simulink model "Project_Mobius"  (R2023b)
settings: Solver=ode4  StartTime=0.0  StopTime=100  FixedStep=5e-3  RelTol=1e-3
values from neighbouring files (symbols this model uses):
  aileron_stuck = 0.1    [fault_insertion.m]
  aircraft_b = 2    [initial.m]
  aircraft_c = 0.275    [initial.m]
  aircraft_mass = 6.031    [initial.m]
  c1 = ((Iyy - Izz)*Izz - Ixz*Ixz)/sigma    (= -0.404494382022)    [initial.m]
  c2 = ((Ixx - Iyy + Izz)*Ixz)/sigma    (= 0)    [initial.m]
  c3 = Izz/sigma    (= 3.74531835206)    [initial.m]
  c4 = Ixz/sigma    (= 0)    [initial.m]
  c5 = (Izz - Ixx)/Iyy    (= 0.404494382022)    [initial.m]
  c6 = Ixz/Iyy    (= 0)    [initial.m]
  c7 = 1/Iyy    (= 3.74531835206)    [initial.m]
  c8 = (Ixx*(Ixx - Iyy) + Ixz*Ixz)/sigma    (= 0)    [initial.m]
  c9 = Ixx/sigma    (= 2.66666666667)    [initial.m]
  CD_fuselage = 0.027    [initial.m]
  CdDa = 0.092132    [initial.m]
  CdDe = 0.016043    [initial.m]
  CdDr = 0.0097403    [initial.m]
  CDmin = 0.06047    [initial.m]
  CL0 = 0.81857    [initial.m]
  CL_CDmin = 0.4806    [initial.m]
  CLa = 4.09127    [initial.m]
  CLa_dot = 0    [initial.m]
  Clb = -0.00161    [initial.m]
  ClDa = 0.286593    [initial.m]
  CLDa = -0.85291    [initial.m]
  CLDe = 0.50787    [initial.m]
  ClDr = 0.013407    [initial.m]
  Clp = -0.47584    [initial.m]
  CLq = 7.31097    [initial.m]
  Clr = 0.27153    [initial.m]
  Cm0 = 0.00763    [initial.m]
  Cma = -1.76966    [initial.m]
  CmDe = -1.83747    [initial.m]
  Cmq = -19.22663    [initial.m]
  Cnb = 0.0918    [initial.m]
  CnDa = 0.0049274    [initial.m]
  CnDr = -0.067036    [initial.m]
  Cnp = -0.13267    [initial.m]
  Cnr = -0.08829    [initial.m]
  CYb = -0.00157    [initial.m]
  CYDr = 0.128915    [initial.m]
  CYp = -0.00157    [initial.m]
  CYr = 0.18368    [initial.m]
  elevator_stuck = 0    [fault_insertion.m]
  fault_time_start = 1    [fault_insertion.m]
  flight_mode = 1    [initial.m]
  g = 9.8060    (= 9.806)    [initial.m]
  init_alpha = alpha_trim    (= 0)    [initial.m]
  init_h = 10    [initial.m]
  init_p = 0    [initial.m]
  init_phi = 0    [initial.m]
  init_psi = 0    [initial.m]
  init_q = 0    [initial.m]
  init_r = 0    [initial.m]
  init_theta = init_alpha    (= 0)    [initial.m]
  init_u = Vb(1)    [initial.m]
  init_v = Vb(2)    [initial.m]
  init_w = Vb(3)    [initial.m]
  init_x = 0    [initial.m]
  init_y = 0    [initial.m]
  K = 0.1328    [initial.m]
  Max_RPM = 10000    [initial.m]
  p_sensor_fault = 0    [fault_insertion.m]
  phi_sensor_fault = 0    [fault_insertion.m]
  PropDiameter = 0.3052    [initial.m]
  psi_sensor_fault = 0    [fault_insertion.m]
  q_sensor_fault = 0    [fault_insertion.m]
  r_sensor_fault = 0    [fault_insertion.m]
  rho = 1.2250    (= 1.225)    [initial.m]
  rotor1_direction = 1    [initial.m]
  rotor1_fail = 0    [fault_insertion.m]
  rotor2_direction = -1    [initial.m]
  rotor2_fail = 0    [fault_insertion.m]
  rotor3_direction = -1    [initial.m]
  rotor3_fail = 0    [fault_insertion.m]
  rotor4_direction = 1    [initial.m]
  rotor4_fail = 0    [fault_insertion.m]
  rotor_arm1 = [0.375,0.375,0]    [initial.m]
  rotor_arm2 = [0.375,-0.375,0]    [initial.m]
  rotor_arm3 = [-0.375,-0.375,0]    [initial.m]
  rotor_arm4 = [-0.375,0.375,0]    [initial.m]
  RPM1_init = rotor_n * 60    (= 5940)    [initial.m]
  RPM2_init = rotor_n * 60    (= 5940)    [initial.m]
  RPM3_init = 0    [initial.m]
  RPM4_init = 0    [initial.m]
  rudder_stuck = 0    [fault_insertion.m]
  theta_sensor_fault = 0    [fault_insertion.m]
  tilt1_fail = 0    [fault_insertion.m]
  tilt1_init = lambda    [initial.m]
  tilt2_fail = 0    [fault_insertion.m]
  tilt2_init = lambda    [initial.m]
  tilt3_init = 0    [initial.m]
  tilt4_init = 0    [initial.m]
  u_sensor_fault = 0    [fault_insertion.m]
  v_sensor_fault = 0    [fault_insertion.m]
  w_sensor_fault = 0    [fault_insertion.m]
undefined symbols (not defined in the file or in its folder): FixedWingMission, HoverMission
libraries: slpidlib x20, simulink_extras x12, simulink x7, aerolibasang x6, matrix_library x4, uavalgslib x4, sharedutil x1, sharedtransform x1
(part 4 of 4)

== system Project_Mobius/EVTOL Model/6DOF Dynamics/Subsystem ==
  In2 : Inport  Unit=rad  PortDimensions=3
  Create 3x3 Matrix : sharedutil/Create 3x3 Matrix  aMode=aMode
  Dead Zone : DeadZone  LowerValue=-cos(pi/2)  UpperValue=cos(pi/2)
  Fcn11 : Fcn  Expr=u(5)*u(4)
  Fcn12 : Fcn  Expr=u(5)*u(1)
  Fcn13 : Fcn  Expr=-u(2)
  Fcn21 : Fcn  Expr=u(3)*u(2)*u(4) - u(6)*u(1)
  Fcn22 : Fcn  Expr=u(3)*u(2)*u(1) + u(6)*u(4)
  Fcn23 : Fcn  Expr=u(3)*u(5)
  Fcn31 : Fcn  Expr=u(6)*u(2)*u(4) + u(3)*u(1)
  Fcn32 : Fcn  Expr=u(6)*u(2)*u(1) - u(3)*u(4)
  Fcn33 : Fcn  Expr=u(6)*u(5)
  Mux : Mux  Inputs=2
  sincos : Trigonometry  Operator=sincos
  DCMbe : Outport  Unit=1  PortDimensions=[3,3]  VectorParamsAs1DForOutWhenUnconnected=off
  wires:
  Fcn23/1 -> Create 3x3 Matrix/6
  Fcn31/1 -> Create 3x3 Matrix/7
  sincos/2 -> Dead Zone/1
  Fcn22/1 -> Create 3x3 Matrix/5
  Fcn21/1 -> Create 3x3 Matrix/4
  Fcn32/1 -> Create 3x3 Matrix/8
  Fcn33/1 -> Create 3x3 Matrix/9
  Mux/1 -> Fcn11/1, Fcn12/1, Fcn13/1, Fcn21/1, Fcn32/1, Fcn33/1, Fcn31/1, Fcn23/1, Fcn22/1
  In2/1 -> sincos/1
  Create 3x3 Matrix/1 -> DCMbe/1
  Fcn12/1 -> Create 3x3 Matrix/2
  sincos/1 -> Mux/1
  Fcn13/1 -> Create 3x3 Matrix/3
  Fcn11/1 -> Create 3x3 Matrix/1
  Dead Zone/1 -> Mux/2

== system Project_Mobius/EVTOL Model/Aerodynamic/Lateral ==
  aileron : Inport
  rudder : Inport  Port=2
  V : Inport  Port=3
  pqr : Inport  Port=4
  beta : Inport  Port=5
  Coff_CY : Subsystem
  Coff_Cl : Subsystem
  Subsystem : Subsystem
  CY : Outport
  Cl : Outport  Port=2
  Cn : Outport  Port=3
  wires:
  beta/1 -> Subsystem/1(beta), Coff_Cl/1(beta), Coff_CY/1(beta)
  rudder/1 -> Coff_Cl/3(rudder), Subsystem/3(rudder), Coff_CY/2(Rudder)
  pqr/1 -> Subsystem/4(pqr), Coff_Cl/5(pqr), Coff_CY/3(pqr)
  V/1 -> Subsystem/5(V), Coff_Cl/4(V), Coff_CY/4(V)
  Coff_CY/1(CY) -> CY/1
  aileron/1 -> Subsystem/2(aileron), Coff_Cl/2(aileron)
  Coff_Cl/1(Cl) -> Cl/1
  Subsystem/1(Cn) -> Cn/1

== system Project_Mobius/EVTOL Model/Aerodynamic/Longitudinal ==
  alpha : Inport
  V : Inport  Port=2
  elevator : Inport  Port=3
  pqr : Inport  Port=4
  aileron : Inport  Port=5
  rudder : Inport  Port=6
  Coff_D : Subsystem
  Coff_L : Subsystem
  Gain : Gain  Gain=-1
  Saturation : Saturate  UpperLimit=14*pi/180  LowerLimit=-14*pi/180
  Subsystem : Subsystem
  Transfer Fcn : TransferFcn  Numerator=[1 0]  Denominator=[0.1 1]
  CD : Outport
  CL : Outport  Port=2
  Cm : Outport  Port=3
  wires:
  aileron/1 -> Coff_L/6(aileron), Coff_D/2(aileron)
  rudder/1 -> Coff_D/3(rudder)
  elevator/1 -> Subsystem/2(elevator), Coff_L/3(elevator), Coff_D/4(elevator)
  Coff_D/1(CD) -> CD/1
  alpha/1 -> Saturation/1
  Saturation/1 -> Transfer Fcn/1, Subsystem/1(alpha), Coff_L/1(alpha)
  Transfer Fcn/1 -> Coff_L/2(alpha_dot)
  pqr/1 -> Subsystem/3(pqr), Coff_L/4(pqr)
  V/1 -> Subsystem/4(V), Coff_L/5(V)
  Coff_L/1(CL) -> Coff_D/1(CL), Gain/1
  Subsystem/1(Cm) -> Cm/1
  Gain/1 -> CL/1

== system Project_Mobius/EVTOL Model/Rotors/Rotor1_Dynamics ==
  throttle : Inport
  V : Inport  Port=2
  CQ : Polyval  Coefs=[0.04280,-0.05046,0.005711,-0.003293, 0.007048]
  CT : Polyval  Coefs=[0.03338, -0.1265,-0.1210,0.1142]
  Constant : Constant  Value=PropDiameter
  Constant1 : Constant  Value=rho
  Constant2 : Constant  Value=4
  Constant3 : Constant  Value=5
  Divide : Product  Inputs=*/
  Gain : Gain  Gain=1/60
  Gain1 : Gain  Gain=Max_RPM
  Power : Math  Operator=pow
  Power1 : Math  Operator=pow
  Product : Product  Inputs=4
  Product1 : Product  Inputs=4
  Product2 : Product
  Saturation : Saturate  UpperLimit=1  LowerLimit=0.1
  Scope : Scope
  Scope1 : Scope
  Square : Math  Operator=square
  Transfer Fcn (with initial outputs)1 : simulink_extras/Additional Linear/Transfer Fcn (with initial outputs)  N=[1]  D="[0.02  1]"  Y0=RPM1_init  U0=RPM1_init
  F_rotor : Outport
  M_rotor : Outport  Port=2
  w1 : Outport  Port=3
  wires:
  Saturation/1 -> Gain1/1
  throttle/1 -> Saturation/1
  Constant/1 -> Power1/1, Power/1, Product2/1
  Gain1/1 -> Scope/1, Transfer Fcn (with initial outputs)1/1
  Product2/1 -> Divide/2
  V/1 -> Divide/1
  Divide/1 -> CQ/1, CT/1
  Constant2/1 -> Power/2
  Power/1 -> Product/1
  Constant1/1 -> Product1/2, Product/2
  CT/1 -> Product/3
  Square/1 -> Product1/4, Product/4
  Product/1 -> F_rotor/1
  CQ/1 -> Product1/1
  Power1/1 -> Product1/3
  Constant3/1 -> Power1/2
  Product1/1 -> M_rotor/1
  Transfer Fcn (with initial outputs)1/1 -> Scope1/1, Gain/1
  Gain/1 -> w1/1, Square/1, Product2/2

== system Project_Mobius/EVTOL Model/Rotors/Rotor2_Dynamics ==
  V : Inport
  throttle : Inport  Port=2
  CQ : Polyval  Coefs=[0.04280,-0.05046,0.005711,-0.003293, 0.007048]
  CT : Polyval  Coefs=[0.03338, -0.1265,-0.1210,0.1142]
  Constant : Constant  Value=PropDiameter
  Constant1 : Constant  Value=rho
  Constant2 : Constant  Value=4
  Constant3 : Constant  Value=5
  Divide : Product  Inputs=*/
  Gain : Gain  Gain=1/60
  Gain1 : Gain  Gain=Max_RPM
  Power : Math  Operator=pow
  Power1 : Math  Operator=pow
  Product : Product  Inputs=4
  Product1 : Product  Inputs=4
  Product2 : Product
  Saturation : Saturate  UpperLimit=1  LowerLimit=0.1
  Square : Math  Operator=square
  Transfer Fcn (with initial outputs)1 : simulink_extras/Additional Linear/Transfer Fcn (with initial outputs)  N=[1]  D="[0.02  1]"  Y0=RPM2_init  U0=RPM2_init
  F_rotor : Outport
  M_rotor : Outport  Port=2
  w2 : Outport  Port=3
  wires:
  Saturation/1 -> Gain1/1
  throttle/1 -> Saturation/1
  Constant/1 -> Power1/1, Power/1, Product2/1
  Gain1/1 -> Transfer Fcn (with initial outputs)1/1
  Product2/1 -> Divide/2
  V/1 -> Divide/1
  Divide/1 -> CQ/1, CT/1
  Constant2/1 -> Power/2
  Power/1 -> Product/1
  Constant1/1 -> Product1/2, Product/2
  CT/1 -> Product/3
  Square/1 -> Product1/4, Product/4
  Product/1 -> F_rotor/1
  CQ/1 -> Product1/1
  Power1/1 -> Product1/3
  Constant3/1 -> Power1/2
  Product1/1 -> M_rotor/1
  Transfer Fcn (with initial outputs)1/1 -> Gain/1
  Gain/1 -> w2/1, Square/1, Product2/2

== system Project_Mobius/EVTOL Model/Rotors/Rotor3_Dynamics ==
  V : Inport
  throttle : Inport  Port=2
  Enable : EnablePort
  CQ : Polyval  Coefs=[0.04280,-0.05046,0.005711,-0.003293, 0.007048]
  CT : Polyval  Coefs=[0.03338, -0.1265,-0.1210,0.1142]
  Constant : Constant  Value=PropDiameter
  Constant1 : Constant  Value=rho
  Constant2 : Constant  Value=4
  Constant3 : Constant  Value=5
  Divide : Product  Inputs=*/
  Gain : Gain  Gain=1/60
  Gain1 : Gain  Gain=Max_RPM
  Power : Math  Operator=pow
  Power1 : Math  Operator=pow
  Product : Product  Inputs=4
  Product1 : Product  Inputs=4
  Product2 : Product
  Saturation : Saturate  UpperLimit=1  LowerLimit=0.1
  Square : Math  Operator=square
  Transfer Fcn (with initial outputs)1 : simulink_extras/Additional Linear/Transfer Fcn (with initial outputs)  N=[1]  D="[0.02  1]"  Y0=RPM3_init  U0=RPM3_init
  F_rotor : Outport
  M_rotor : Outport  Port=2
  w3 : Outport  Port=3
  wires:
  Saturation/1 -> Gain1/1
  throttle/1 -> Saturation/1
  Constant/1 -> Power1/1, Power/1, Product2/1
  Gain1/1 -> Transfer Fcn (with initial outputs)1/1
  Product2/1 -> Divide/2
  V/1 -> Divide/1
  Divide/1 -> CQ/1, CT/1
  Constant2/1 -> Power/2
  Power/1 -> Product/1
  Constant1/1 -> Product1/2, Product/2
  CT/1 -> Product/3
  Square/1 -> Product1/4, Product/4
  Product/1 -> F_rotor/1
  CQ/1 -> Product1/1
  Power1/1 -> Product1/3
  Constant3/1 -> Power1/2
  Product1/1 -> M_rotor/1
  Transfer Fcn (with initial outputs)1/1 -> Gain/1
  Gain/1 -> w3/1, Square/1, Product2/2

== system Project_Mobius/EVTOL Model/Rotors/Rotor4_Dynamics ==
  V : Inport
  throttle : Inport  Port=2
  Enable : EnablePort
  CQ : Polyval  Coefs=[0.04280,-0.05046,0.005711,-0.003293, 0.007048]
  CT : Polyval  Coefs=[0.03338, -0.1265,-0.1210,0.1142]
  Constant : Constant  Value=PropDiameter
  Constant1 : Constant  Value=rho
  Constant2 : Constant  Value=4
  Constant3 : Constant  Value=5
  Divide : Product  Inputs=*/
  Gain : Gain  Gain=1/60
  Gain1 : Gain  Gain=Max_RPM
  Power : Math  Operator=pow
  Power1 : Math  Operator=pow
  Product : Product  Inputs=4
  Product1 : Product  Inputs=4
  Product2 : Product
  Saturation : Saturate  UpperLimit=1  LowerLimit=0.1
  Square : Math  Operator=square
  Transfer Fcn (with initial outputs)1 : simulink_extras/Additional Linear/Transfer Fcn (with initial outputs)  N=[1]  D="[0.02  1]"  Y0=RPM4_init  U0=RPM4_init
  F_rotor : Outport
  M_rotor : Outport  Port=2
  w4 : Outport  Port=3
  wires:
  Saturation/1 -> Gain1/1
  throttle/1 -> Saturation/1
  Constant/1 -> Power1/1, Power/1, Product2/1
  Gain1/1 -> Transfer Fcn (with initial outputs)1/1
  Product2/1 -> Divide/2
  V/1 -> Divide/1
  Divide/1 -> CQ/1, CT/1
  Constant2/1 -> Power/2
  Power/1 -> Product/1
  Constant1/1 -> Product1/2, Product/2
  CT/1 -> Product/3
  Square/1 -> Product1/4, Product/4
  Product/1 -> F_rotor/1
  CQ/1 -> Product1/1
  Power1/1 -> Product1/3
  Constant3/1 -> Power1/2
  Product1/1 -> M_rotor/1
  Transfer Fcn (with initial outputs)1/1 -> Gain/1
  Gain/1 -> w4/1, Square/1, Product2/2

== system Project_Mobius/Guidance/Guidance Command/Attitude Stablizer ==
  Mux : Mux  Inputs=2
  Pitch : Constant  Value=0
  Roll : Constant  Value=0
  Attitude : Outport
  wires:
  Roll/1 -> Mux/1
  Pitch/1 -> Mux/2
  Mux/1 -> Attitude/1

== system Project_Mobius/Guidance/Guidance Command/Path_selector ==
  courseSP : Inport
  positionSP : Inport  Port=2
  Mux : Mux  Inputs=2
  Xe_cmd : Outport
  wires:
  Mux/1 -> Xe_cmd/1
  courseSP/1 -> Mux/2
  positionSP/1 -> Mux/1

== system Project_Mobius/Guidance/MultiRotor Mode/Dist2WP ==
  FromWP : Inport
  ToWP : Inport  Port=2
  Pose : Inport  Port=3
  Bus Selector : BusSelector  OutputSignals=position
  Bus Selector1 : BusSelector  OutputSignals=position
  Demux : Demux  Outputs=[3 1]
  Dot Product : DotProduct  OutDataTypeStr=Inherit: Inherit via internal rule
  Subsystem : Subsystem
  Sum : Sum  Inputs=|-+
  Sum1 : Sum  Inputs=|+-
  Terminator : Terminator
  Dist : Outport
  wires:
  Sum1/1 -> Subsystem/1(V)
  Demux/2 -> Terminator/1
  Bus Selector/1 -> Sum/2, Sum1/1  "<position>"
  Demux/1 -> Sum/1
  Bus Selector1/1 -> Sum1/2  "<position>"
  Sum/1 -> Dot Product/1
  Subsystem/1(V_unit) -> Dot Product/2
  Pose/1 -> Demux/1
  Dot Product/1 -> Dist/1
  ToWP/1 -> Bus Selector/1
  FromWP/1 -> Bus Selector1/1

== system Project_Mobius/AutoPilot/Fixed-Wing/Attitude Controller/Turn Coordinator ==
  Roll SP : Inport
  Pitch SP : Inport  Port=2
  Airspeed : Inport  Port=3
  r : Inport  Port=4
  MATLAB Function : MATLAB Function  TreatAsAtomicUnit=on
  Rudder Controller : slpidlib/PID Controller  Controller=P  Form=Parallel  TimeDomain=Continuous-time  UseExternalTs=off  SampleTime=-1  IntegratorMethod=Forward Euler  FilterMethod=Forward Euler  ControllerParametersSource=internal  P=0.01  I=1  UseKiTs=off  D=0  N=100  UseFilter=on  TunerSelectOption=Transfer Function Based (PID Tuner App)  InitialConditionSource=internal  InitialConditionForIntegrator=0  InitialConditionForFilter=0  DifferentiatorICPrevScaledInput=0  ExternalReset=none  TrackingMode=off  Kt=1  LimitOutput=on  SatLimitsSource=internal  UpperSaturationLimit=1  LowerSaturationLimit=-1  LinearizeAsGain=on  AntiWindupMode=none  Kb=1  LimitIntegrator=off  UpperIntegratorSaturationLimit=inf  LowerIntegratorSaturationLimit=-inf  POutMin=[]  POutMax=[]  IOutMin=[]  IOutMax=[]  DOutMin=[]  DOutMax=[]  NOutMin=[]  NOutMax=[]  SumOutMin=[]  SumOutMax=[]  SaturationOutMin=[]  SaturationOutMax=[]  PParamMin=[]  PParamMax=[]  IParamMin=[]  IParamMax=[]  DParamMin=[]  DParamMax=[]  NParamMin=[]  NParamMax=[]  KbParamMin=[]  KbParamMax=[]  KtParamMin=[]  KtParamMax=[]  KbOutMin=[]  KbOutMax=[]  KtOutMin=[]  KtOutMax=[]  IntegratorOutMin=[]  IntegratorOutMax=[]  FilterOutMin=[]  FilterOutMax=[]  SumI1OutMin=[]  SumI1OutMax=[]  SumI2OutMin=[]  SumI2OutMax=[]  SumI3OutMin=[]  SumI3OutMax=[]  SumI4OutMin=[]  SumI4OutMax=[]  SumDOutMin=[]  SumDOutMax=[]  DifferentiatorOutMin=[]  DifferentiatorOutMax=[]  FilterDiffOutCoefMin=[]  FilterDiffOutCoefMax=[]  ReciprocalOutMin=[]  ReciprocalOutMax=[]  SumDenOutMin=[]  SumDenOutMax=[]  SumNumOutMin=[]  SumNumOutMax=[]  DivideOutMin=[]  DivideOutMax=[]  UdiffTsProdOutMin=[]  UdiffTsProdOutMax=[]  NTsProdOutMin=[]  NTsProdOutMax=[]  UintegralTsProdOutMin=[]  UintegralTsProdOutMax=[]  UngainTsProdOutMin=[]  UngainTsProdOutMax=[]  ClampingZeroOutDataTypeStr=Inherit: Inherit via back propagation  ClampingZeroOutMin=[]  ClampingZeroOutMax=[]  FilterDenConstantOutDataTypeStr=Inherit: Inherit via back propagation  FilterDenConstantOutMin=[]  FilterDenConstantOutMax=[]  PCopyOutDataTypeStr=Inherit: Inherit via back propagation  PCopyOutMin=[]  PCopyOutMax=[]  NCopyOutDataTypeStr=Inherit: Inherit via back propagation  NCopyOutMin=[]  NCopyOutMax=[]  IntegratorContinuousStateAttributes=''  IntegratorStateMustResolveToSignalObject=off  IntegratorRTWStateStorageClass=Auto  FilterContinuousStateAttributes=''  FilterStateMustResolveToSignalObject=off  FilterRTWStateStorageClass=Auto  ParallelPVariant=InternalParameters  IdealPVariant=Disabled  IVariant=Disabled  DVariant=Disabled  IntegratorVariant=Disabled  SatVariant=Enabled  AWVariant=Disabled  PCopyVariant=Disabled  TRVariant=Disabled  FdbkBlocksVariant=Forward  IdealPFdbkVariant=Disabled  SatFdbkVariant=Disabled  DerivativeFilterVariant=Disabled  NVariant=Disabled  NCopyVariant=Disabled_SignalSpec  FilterICVariant=Disabled  IntegratorICVariant=Disabled  ExternalResetVariant=Disabled  TRSumVariant=Passthrough  SumFdbkVariant=Disabled  SumVariant=Passthrough_P  TsampFilterVariant=InternalTs  TsampNgainVariant=Passthrough  TsampIntegralVariant=Disabled_SignalSpec  ExternalSaturationOutDataTypeStr=Inherit: Same as second input
  Sum : Sum  Inputs=|+-
  Rudder : Outport
  wires:
  Roll SP/1 -> MATLAB Function/1(rollSP)
  Pitch SP/1 -> MATLAB Function/2(pitchSP)
  Airspeed/1 -> MATLAB Function/3(airSpeed)
  Sum/1 -> Rudder Controller/1
  Rudder Controller/1 -> Rudder/1
  r/1 -> Sum/2  "r"
  MATLAB Function/1(rSP) -> Sum/1  "rSP"

== system Project_Mobius/EVTOL Model/Aerodynamic/Lateral/Coff_CY ==
  beta : Inport
  Rudder : Inport  Port=2
  pqr : Inport  Port=3
  V : Inport  Port=4
  Add : Sum  Inputs=++++
  CYDr : Constant  Value=CYDr
  CYb : Constant  Value=CYb
  Product : Product
  Product1 : Product
  roll/yaw factors : Subsystem
  CY : Outport
  wires:
  CYb/1 -> Product/1
  beta/1 -> Product/2
  Add/1 -> CY/1
  Product/1 -> Add/1
  Rudder/1 -> Product1/1
  CYDr/1 -> Product1/2
  Product1/1 -> Add/2
  pqr/1 -> roll/yaw factors/1(pqr)
  V/1 -> roll/yaw factors/2(V)
  roll/yaw factors/1(CYp) -> Add/3
  roll/yaw factors/2(CYr) -> Add/4

== system Project_Mobius/EVTOL Model/Aerodynamic/Lateral/Coff_Cl ==
  beta : Inport
  aileron : Inport  Port=2
  rudder : Inport  Port=3
  V : Inport  Port=4
  pqr : Inport  Port=5
  Add : Sum  Inputs=+++++
  ClDa : Constant  Value=ClDa
  ClDr : Constant  Value=ClDr
  Clb : Constant  Value=Clb
  Product : Product
  Product1 : Product
  Product2 : Product
  roll/yaw factors : Subsystem
  Cl : Outport
  wires:
  beta/1 -> Product/2
  Clb/1 -> Product/1
  Product/1 -> Add/1
  ClDa/1 -> Product1/1
  aileron/1 -> Product1/2
  ClDr/1 -> Product2/1
  rudder/1 -> Product2/2
  Product1/1 -> Add/2
  Product2/1 -> Add/3
  pqr/1 -> roll/yaw factors/1(pqr)
  V/1 -> roll/yaw factors/2(V)
  roll/yaw factors/1(Clp) -> Add/4
  roll/yaw factors/2(Clr) -> Add/5
  Add/1 -> Cl/1

== system Project_Mobius/EVTOL Model/Aerodynamic/Lateral/Subsystem ==
  beta : Inport
  aileron : Inport  Port=2
  rudder : Inport  Port=3
  pqr : Inport  Port=4
  V : Inport  Port=5
  Add : Sum  Inputs=+++++
  CnDa : Constant  Value=CnDa
  CnDr : Constant  Value=CnDr
  Cnb : Constant  Value=Cnb
  Product : Product
  Product1 : Product
  Product2 : Product
  roll/yaw factors : Subsystem
  Cn : Outport
  wires:
  beta/1 -> Product/2
  Cnb/1 -> Product/1
  aileron/1 -> Product1/2
  CnDa/1 -> Product1/1
  rudder/1 -> Product2/2
  CnDr/1 -> Product2/1
  Product/1 -> Add/1
  Product1/1 -> Add/2
  Product2/1 -> Add/3
  Add/1 -> Cn/1
  pqr/1 -> roll/yaw factors/1(pqr)
  V/1 -> roll/yaw factors/2(V)
  roll/yaw factors/1(Cnp) -> Add/4
  roll/yaw factors/2(Cnr) -> Add/5

== system Project_Mobius/EVTOL Model/Aerodynamic/Longitudinal/Coff_D ==
  CL : Inport
  aileron : Inport  Port=2
  rudder : Inport  Port=3
  elevator : Inport  Port=4
  Abs : Abs  SaturateOnIntegerOverflow=off
  Abs1 : Abs  SaturateOnIntegerOverflow=off
  Abs2 : Abs  SaturateOnIntegerOverflow=off
  Add : Sum
  Add1 : Sum  Inputs=+-
  Add2 : Sum  Inputs=++++
  CDmin : Constant  Value=CDmin
  CL_CDmin : Constant  Value=CL_CDmin
  CdDa : Constant  Value=CdDa
  CdDe : Constant  Value=CdDe
  CdDr : Constant  Value=CdDr
  Constant1 : Constant  Value=K
  Gain : Gain  Gain=-1
  Product{,2..4} (4 alike) : Product
  Square : Math  Operator=square
  CD : Outport
  wires:
  CDmin/1 -> Add/1
  CL/1 -> Add1/1
  CL_CDmin/1 -> Add1/2
  Add1/1 -> Square/1
  Square/1 -> Product/2
  Constant1/1 -> Product/1
  Product/1 -> Add/2
  Add/1 -> Add2/1
  aileron/1 -> Abs/1
  Abs/1 -> Product2/1
  CdDa/1 -> Product2/2
  Product2/1 -> Add2/2
  Abs1/1 -> Product3/1
  rudder/1 -> Abs1/1
  CdDr/1 -> Product3/2
  elevator/1 -> Abs2/1
  Abs2/1 -> Product4/1
  CdDe/1 -> Product4/2
  Product3/1 -> Add2/3
  Product4/1 -> Add2/4
  Add2/1 -> Gain/1
  Gain/1 -> CD/1

== system Project_Mobius/EVTOL Model/Aerodynamic/Longitudinal/Coff_L ==
  alpha : Inport
  alpha_dot : Inport  Port=2
  elevator : Inport  Port=3
  pqr : Inport  Port=4
  V : Inport  Port=5
  aileron : Inport  Port=6
  Abs : Abs  SaturateOnIntegerOverflow=off
  Add : Sum  Inputs=++++++
  CL0 : Constant  Value=CL0
  CLDa : Constant  Value=CLDa
  CLDe : Constant  Value=CLDe
  CLa : Constant  Value=CLa
  CLa_dot : Constant  Value=CLa_dot
  CLq : Constant  Value=CLq
  Demux : Demux  Outputs=3
  Gain : Gain  Gain=2
  Product{,1..3,5} (5 alike) : Product
  Product4 : Product  Inputs=**/
  Saturation : Saturate  UpperLimit=inf  LowerLimit=0.1
  c : Constant  Value=aircraft_c
  CL : Outport
  wires:
  alpha/1 -> Product/2
  CLa/1 -> Product/1
  CL0/1 -> Add/1
  Product/1 -> Add/2
  CLa_dot/1 -> Product1/1
  alpha_dot/1 -> Product1/2
  Product1/1 -> Add/3
  elevator/1 -> Product2/2
  CLDe/1 -> Product2/1
  Product2/1 -> Add/4
  CLDa/1 -> Product3/1
  Product3/1 -> Add/5
  aileron/1 -> Abs/1
  Abs/1 -> Product3/2
  pqr/1 -> Demux/1
  Demux/2 -> Product4/1
  c/1 -> Product4/2
  V/1 -> Saturation/1
  Saturation/1 -> Gain/1
  Gain/1 -> Product4/3
  CLq/1 -> Product5/1
  Product4/1 -> Product5/2
  Product5/1 -> Add/6
  Add/1 -> CL/1

== system Project_Mobius/EVTOL Model/Aerodynamic/Longitudinal/Subsystem ==
  alpha : Inport
  elevator : Inport  Port=2
  pqr : Inport  Port=3
  V : Inport  Port=4
  Add : Sum  Inputs=++++
  Cm0 : Constant  Value=Cm0
  CmDe : Constant  Value=CmDe
  Cma : Constant  Value=Cma
  Cmq : Constant  Value=Cmq
  Demux : Demux  Outputs=3
  Gain : Gain  Gain=2
  Product : Product
  Product1 : Product
  Product4 : Product  Inputs=**/
  Product5 : Product
  Saturation : Saturate  UpperLimit=inf  LowerLimit=0.1
  c : Constant  Value=aircraft_c
  Cm : Outport
  wires:
  Cm0/1 -> Add/1
  alpha/1 -> Product/2
  Cma/1 -> Product/1
  Product/1 -> Add/2
  elevator/1 -> Product1/2
  CmDe/1 -> Product1/1
  Product1/1 -> Add/3
  Saturation/1 -> Gain/1
  Cmq/1 -> Product5/1
  Gain/1 -> Product4/3
  V/1 -> Saturation/1
  Product4/1 -> Product5/2
  c/1 -> Product4/2
  Demux/2 -> Product4/1
  pqr/1 -> Demux/1
  Product5/1 -> Add/4
  Add/1 -> Cm/1

== system Project_Mobius/Guidance/MultiRotor Mode/Dist2WP/Subsystem ==
  V : Inport
  Dot Product1 : DotProduct  OutDataTypeStr=Inherit: Inherit via internal rule
  Product : Product  Inputs=*/
  Saturation : Saturate  UpperLimit=inf  LowerLimit=0.00001
  Sqrt : Sqrt
  V_unit : Outport
  wires:
  V/1 -> Dot Product1/2, Dot Product1/1, Product/1
  Sqrt/1 -> Product/2
  Dot Product1/1 -> Saturation/1
  Saturation/1 -> Sqrt/1
  Product/1 -> V_unit/1

== system Project_Mobius/EVTOL Model/Aerodynamic/Lateral/Coff_CY/roll//yaw factors ==
  pqr : Inport
  V : Inport  Port=2
  Cmq : Constant
  Coff_Yp : Constant  Value=CYp
  Coff_Yr : Constant  Value=CYr
  Demux : Demux  Outputs=3
  Gain : Gain  Gain=2
  Product : Product  Inputs=***/
  Product1 : Product
  Product2 : Product  Inputs=***/
  Product3 : Product
  Saturation : Saturate  UpperLimit=inf  LowerLimit=0.1
  b : Constant  Value=aircraft_b
  CYp : Outport
  CYr : Outport  Port=2
  wires:
  pqr/1 -> Demux/1
  Demux/1 -> Product/1
  Cmq/1 -> Product2/2, Product/2
  b/1 -> Product2/3, Product/3
  V/1 -> Saturation/1
  Saturation/1 -> Gain/1
  Gain/1 -> Product2/4, Product/4
  Product1/1 -> CYp/1
  Product/1 -> Product1/2
  Coff_Yp/1 -> Product1/1
  Product2/1 -> Product3/1
  Coff_Yr/1 -> Product3/2
  Demux/3 -> Product2/1
  Product3/1 -> CYr/1

== system Project_Mobius/EVTOL Model/Aerodynamic/Lateral/Coff_Cl/roll//yaw factors ==
  pqr : Inport
  V : Inport  Port=2
  Cmq : Constant  Value=0.5
  Coff_lp : Constant  Value=Clp
  Coff_lr : Constant  Value=Clr
  Demux : Demux  Outputs=3
  Product : Product  Inputs=***/
  Product1 : Product
  Product2 : Product  Inputs=***/
  Product3 : Product
  Saturation : Saturate  UpperLimit=inf  LowerLimit=0.1
  b : Constant  Value=aircraft_b
  Clp : Outport
  Clr : Outport  Port=2
  wires:
  pqr/1 -> Demux/1
  Product/1 -> Product1/2
  Cmq/1 -> Product2/2, Product/2
  b/1 -> Product2/3, Product/3
  Demux/1 -> Product/1
  V/1 -> Saturation/1
  Saturation/1 -> Product2/4, Product/4
  Product1/1 -> Clp/1
  Coff_lp/1 -> Product1/1
  Demux/3 -> Product2/1
  Product2/1 -> Product3/1
  Coff_lr/1 -> Product3/2
  Product3/1 -> Clr/1

== system Project_Mobius/EVTOL Model/Aerodynamic/Lateral/Subsystem/roll//yaw factors ==
  pqr : Inport
  V : Inport  Port=2
  Cmq : Constant  Value=0.5
  Coff_np : Constant  Value=Cnp
  Coff_nr : Constant  Value=Cnr
  Demux : Demux  Outputs=3
  Product : Product  Inputs=***/
  Product1 : Product
  Product2 : Product  Inputs=***/
  Product3 : Product
  Saturation : Saturate  UpperLimit=inf  LowerLimit=0.1
  b : Constant  Value=aircraft_b
  Cnp : Outport
  Cnr : Outport  Port=2
  wires:
  pqr/1 -> Demux/1
  Product/1 -> Product1/2
  Cmq/1 -> Product2/2, Product/2
  b/1 -> Product2/3, Product/3
  Demux/1 -> Product/1
  V/1 -> Saturation/1
  Saturation/1 -> Product2/4, Product/4
  Product1/1 -> Cnp/1
  Coff_np/1 -> Product1/1
  Demux/3 -> Product2/1
  Product2/1 -> Product3/1
  Coff_nr/1 -> Product3/2
  Product3/1 -> Cnr/1

== matlab function Project_Mobius/EVTOL Model/MATLAB Function1 ==
  data: vxyz input; course output; gndSpeed output
function [course, gndSpeed] = fcn(vxyz)

vx = vxyz(1);
vy = vxyz(2);
course = atan2(vy, vx);
gndSpeed = norm([vx vy 0]);

== matlab function Project_Mobius/AutoPilot/Fixed-Wing/Position Controller/MATLAB Function ==
  data: courseSP input; lacc output; course input; rollSP output; groundSpeed input; L1 input
function [lacc, rollSP] = fcn(courseSP, course, groundSpeed, L1)
eta = courseSP - course;

% wrap -pi to pi
eta = mod(eta, 2*pi);
if eta>pi
    eta = eta - 2*pi;
end

% cap eta to -pi/2 to pi/2
eta = min(eta, pi/2);
eta = max(eta, -pi/2);

lacc = 2*(groundSpeed^2)/L1*sin(eta);

rollSP = atan(lacc/9.81);

== matlab function Project_Mobius/AutoPilot/Multirotor/MATLAB Function ==
  data: xcmd input; ucmd output; ycmd input; yaw input; vcmd output
function [ucmd,vcmd] = fcn(xcmd,ycmd,yaw)
%xcmd acceleration in NED X direction
ucmd=xcmd*cos(yaw)+ycmd*sin(yaw);
vcmd=-xcmd*sin(yaw)+ycmd*cos(yaw);
end

== matlab function Project_Mobius/Guidance/MultiRotor Mode/MATLAB Function ==
  data: from input; waypoint output; to input
function waypoint = fcn(from,to)

waypoint = [from' 0;to' 0];

== matlab function Project_Mobius/Guidance/Fixed-Wing Mode/MATLAB Function ==
  data: from input; waypoint output; to input
function waypoint = fcn(from,to)

waypoint = [from';to'];

== matlab function Project_Mobius/AutoPilot/Fixed-Wing/Attitude Controller/Turn Coordinator/MATLAB Function ==
  data: rollSP input; rSP output; pitchSP input; airSpeed input
function rSP = fcn(rollSP, pitchSP, airSpeed)
    yawRateSP = tan(rollSP)*9.81/airSpeed;
    rSP = yawRateSP*cos(pitchSP)*cos(rollSP);
end
